simulink model "InverseDynamicsTest"  (R2021b)
settings: Solver=FixedStepAuto  StartTime=0.0  StopTime=5  FixedStep=Ts  RelTol=1e-3
values from neighbouring files (symbols this model uses):
  zdq_A = [1 3*wc 3*wc^2 wc^3]    [search_observer_parameters.m]
  zdq_B = [0 0 0 wc^3]    [search_observer_parameters.m]
undefined symbols (not defined in the file or in its folder): alphas_m, conf, dh, gravity, lambdas_m, x0
libraries: simulink x2, robotcorelib x2, vrlib x1
settings Model: Creator=eros  LastModifiedBy=Sebastiano
settings SolverCC: AlgebraicLoopSolver=TrustRegion
settings DebuggingCC: SFMachineParentedDataDiag=warning

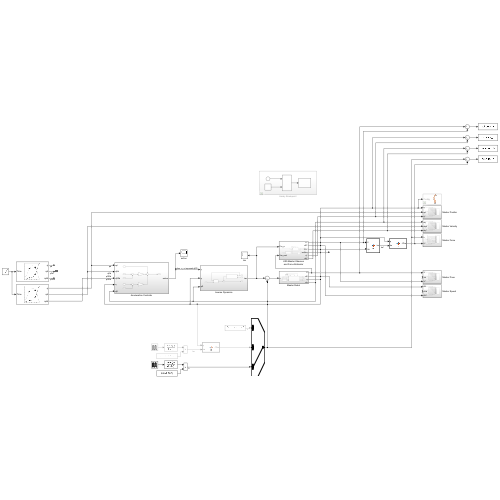
[thumbnail: Simulink's stored preview of the top-level diagram]
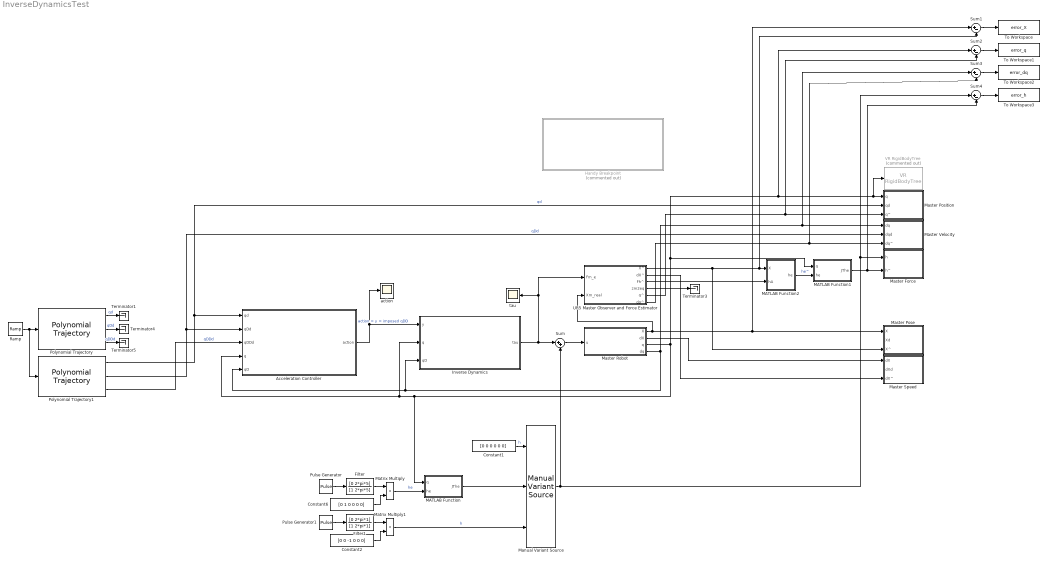
== system InverseDynamicsTest ==
  Acceleration Controller : Subsystem
  Constant1 : Constant  Value=[0 0 0 0 0 0]
  Constant2 : Constant  Value=[0 0 -1 0 0 0]
  Constant6 : Constant  Value=[0 1 0 0 0 0]
  Filter : TransferFcn  Numerator=[0 2*pi*5]  Denominator=[1 2*pi*5]
  Filter1 : TransferFcn  Numerator=[0 2*pi*1]  Denominator=[1 2*pi*1]
  Handy Breakpoint : Subsystem  Commented=on
  Inverse Dynamics : Subsystem
  MATLAB Function : MATLAB Function  TreatAsAtomicUnit=on
  MATLAB Function1 : MATLAB Function  TreatAsAtomicUnit=on
  MATLAB Function2 : MATLAB Function  TreatAsAtomicUnit=on
  Manual Variant Source : simulink/Signal Routing/Manual Variant Source  NumChoices=3  LabelModeActiveChoice=V_3
  Master Force : Subsystem
  Master Pose : Subsystem
  Master Position : Subsystem
  Master Robot : Subsystem
  Master Speed : Subsystem
  Master Velocity : Subsystem
  Matrix Multiply : Product
  Matrix Multiply1 : Product
  Polynomial Trajectory : robotcorelib/Polynomial Trajectory  WaypointSource=Internal  Waypoints=[-1.6007 -1.7271 -2.203 -0.808 1.5951 -0.031; 0 0 0 0 0 0]'  TimePoints=[ 0, 5]  TimeInterval=[ 1, 4 ]  Method=Cubic Polynomial  ParameterSource=Internal  VelocityBoundaryCondition=zeros( 6, 2 )  AccelerationBoundaryCondition=zeros( 2, 5 )  SimulateUsing=Code generation
  Polynomial Trajectory1 : robotcorelib/Polynomial Trajectory  WaypointSource=Internal  Waypoints=[conf.init.q0 conf.init.q0]  TimePoints=[ 0, 5]  TimeInterval=[ 1, 4 ]  Method=Cubic Polynomial  ParameterSource=Internal  VelocityBoundaryCondition=zeros( 6, 2 )  AccelerationBoundaryCondition=zeros( 2, 5 )  SimulateUsing=Code generation
  Pulse Generator : DiscretePulseGenerator  PulseType=Time based  Amplitude=25  Period=3  PulseWidth=50  PhaseDelay=0.5
  Pulse Generator1 : DiscretePulseGenerator  PulseType=Time based  Amplitude=25  Period=3  PulseWidth=50  PhaseDelay=0.5
  Ramp : simulink/Sources/Ramp  slope=1  start=0  InitialOutput=0
  Sum : Sum  Inputs=|++
  Sum{1..4} (4 alike) : Sum  Inputs=|+-
  Terminator{1,3..5} (4 alike) : Terminator
  To Workspace : ToWorkspace  VariableName=error_X  SaveFormat=Timeseries  SampleTime=-1
  To Workspace1 : ToWorkspace  VariableName=error_q  SaveFormat=Timeseries  SampleTime=-1
  To Workspace2 : ToWorkspace  VariableName=error_dq  SaveFormat=Timeseries  SampleTime=-1
  To Workspace3 : ToWorkspace  VariableName=error_h  SaveFormat=Timeseries  SampleTime=-1
  UR5 Master Observer and Force Estimator : Subsystem
  VR RigidBodyTree : vrlib/VR RigidBodyTree  Commented=on  RBT=UR5_robot  useRBT=off  Ts=0.02  ForceViewerOpen=off
      settings: SourceProductBaseCode=SL
  action : Scope
  tau : Scope
  wires:
  Master Robot/4(dq) -> Inverse Dynamics/3(qD), Acceleration Controller/5(qD), Sum3/1, Master Velocity/1(dq)
  Polynomial Trajectory1/3 -> Acceleration Controller/3(qDDd)  "qDDd"
  Inverse Dynamics/1(tau) -> UR5 Master Observer and Force Estimator/1(Fm_e), tau/1, Sum/1
  Polynomial Trajectory1/1 -> Master Position/2(qd), Acceleration Controller/1(qd)  "qd"
  Polynomial Trajectory1/2 -> Master Velocity/2(dqd), Acceleration Controller/2(qDd)  "qDd"
  Acceleration Controller/1(action) -> Inverse Dynamics/1(y), action/1  "action = y = imposed qDD"
  Ramp/1 -> Polynomial Trajectory1/1, Polynomial Trajectory/1
  Sum/1 -> Master Robot/1(u)
  Manual Variant Source/1 -> Sum/2, Sum4/1, Master Force/1(h)
  Pulse Generator/1 -> Filter/1
  Constant6/1 -> Matrix Multiply/2
  Matrix Multiply/1 -> MATLAB Function/2(he)  "he"
  Filter/1 -> Matrix Multiply/1
  UR5 Master Observer and Force Estimator/5(q^) -> Master Position/3(q^), Sum2/2
  UR5 Master Observer and Force Estimator/3(Fh^) -> MATLAB Function2/2(hA)
  UR5 Master Observer and Force Estimator/6(dq^) -> Master Velocity/3(dq^), Sum3/2
  Master Robot/1(X) -> UR5 Master Observer and Force Estimator/2(Xm_real), Sum1/1, Master Pose/1(X)
  Master Robot/2(dX) -> Master Speed/1(dX)
  UR5 Master Observer and Force Estimator/4(zm2eq) -> Terminator3/1
  UR5 Master Observer and Force Estimator/2(dX^) -> Master Speed/3(dX^)
  UR5 Master Observer and Force Estimator/1(X^) -> Master Pose/3(X^), Sum1/2, MATLAB Function2/1(X)
  Constant1/1 -> Manual Variant Source/1  "h"
  MATLAB Function2/1(he) -> MATLAB Function1/2(he)  "he^"
  Master Robot/3(q) -> VR RigidBodyTree/1, Master Position/1(q), Sum2/1, MATLAB Function1/1(q), MATLAB Function/1(q), Acceleration Controller/4(q), Inverse Dynamics/2(q)
  MATLAB Function1/1(JThe) -> Master Force/2(h^), Sum4/2
  MATLAB Function/1(JThe) -> Manual Variant Source/2
  Matrix Multiply1/1 -> Manual Variant Source/3  "h"
  Constant2/1 -> Matrix Multiply1/2
  Filter1/1 -> Matrix Multiply1/1
  Pulse Generator1/1 -> Filter1/1
  Sum1/1 -> To Workspace/1
  Polynomial Trajectory/1 -> Terminator1/1  "qd"
  Polynomial Trajectory/2 -> Terminator4/1  "qDd"
  Polynomial Trajectory/3 -> Terminator5/1  "qDDd"
  Sum2/1 -> To Workspace1/1
  Sum3/1 -> To Workspace2/1
  Sum4/1 -> To Workspace3/1

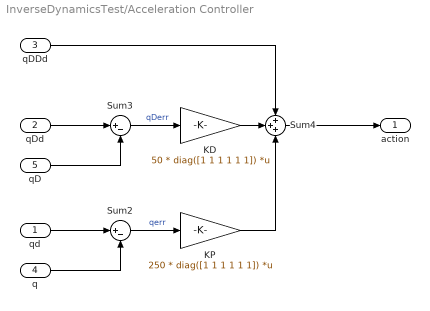
== system InverseDynamicsTest/Acceleration Controller ==
  qd : Inport
  qDd : Inport  Port=2
  qDDd : Inport  Port=3
  q : Inport  Port=4
  qD : Inport  Port=5
  KD : Gain  Gain=50 * diag([1 1 1 1 1 1])  Multiplication=Matrix(K*u) (u vector)
  KP : Gain  Gain=250 * diag([1 1 1 1 1 1])  Multiplication=Matrix(K*u) (u vector)
  Sum2 : Sum  Inputs=|+-
  Sum3 : Sum  Inputs=|+-
  Sum4 : Sum  Inputs=+++
  action : Outport
  wires:
  qDd/1 -> Sum3/1
  KD/1 -> Sum4/2
  KP/1 -> Sum4/3
  qD/1 -> Sum3/2
  Sum3/1 -> KD/1  "qDerr"
  Sum4/1 -> action/1
  Sum2/1 -> KP/1  "qerr"
  qd/1 -> Sum2/1
  qDDd/1 -> Sum4/1
  q/1 -> Sum2/2

== system InverseDynamicsTest/Handy Breakpoint ==
  Assertion : Assertion  AssertionFailFcn=set_param(bdroot,'SimulationCommand','pause')  StopWhenAssertionFail=off
  Clock : Clock
  Constant : Constant  Value=0.5
  Relational Operator : RelationalOperator  Operator=<  OutDataTypeStr=boolean  RndMeth=Simplest
  wires:
  Relational Operator/1 -> Assertion/1
  Constant/1 -> Relational Operator/2
  Clock/1 -> Relational Operator/1

== system InverseDynamicsTest/Inverse Dynamics ==
  y : Inport
  q : Inport  Port=2
  qD : Inport  Port=3
  MATLAB Function : MATLAB Function  TreatAsAtomicUnit=on
  MATLAB Function1 : MATLAB Function  TreatAsAtomicUnit=on
  Sum1 : Sum  Inputs=++|
  tau : Outport
  wires:
  qD/1 -> MATLAB Function/2(qD)
  MATLAB Function/1(n) -> Sum1/1
  MATLAB Function1/1(taud) -> Sum1/2
  q/1 -> MATLAB Function1/1(q), MATLAB Function/1(q)
  y/1 -> MATLAB Function1/2(y)
  Sum1/1 -> tau/1  "tau"

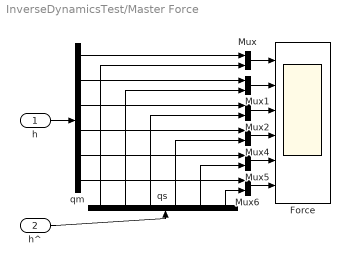
== system InverseDynamicsTest/Master Force ==
  h : Inport
  h^ : Inport  Port=2
  Force : Scope  NumInputPorts=6
  Mux{,1..2,4..6} (6 alike) : Mux  Inputs=2
  qm : Demux  Outputs=dh.dof
  qs : Demux  Outputs=dh.dof
  wires:
  h/1 -> qm/1
  h^/1 -> qs/1
  qm/1 -> Mux/1
  qs/1 -> Mux/2
  qm/2 -> Mux1/1
  qs/2 -> Mux1/2
  qm/3 -> Mux2/1
  qs/3 -> Mux2/2
  qm/4 -> Mux4/1
  qs/4 -> Mux4/2
  Mux/1 -> Force/1
  Mux1/1 -> Force/2
  Mux2/1 -> Force/3
  Mux4/1 -> Force/4
  Mux5/1 -> Force/5
  Mux6/1 -> Force/6
  qs/5 -> Mux5/2
  qm/5 -> Mux5/1
  qm/6 -> Mux6/1
  qs/6 -> Mux6/2

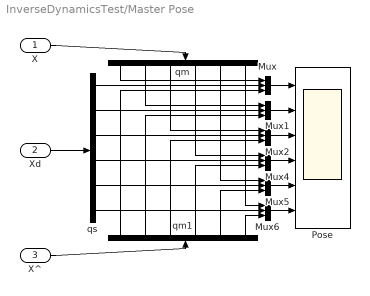
== system InverseDynamicsTest/Master Pose ==
  X : Inport
  Xd : Inport  Port=2
  X^ : Inport  Port=3
  Mux{,1..2,4..6} (6 alike) : Mux  Inputs=3
  Pose : Scope  NumInputPorts=6
  qm : Demux  Outputs=dh.dof
  qm1 : Demux  Outputs=dh.dof
  qs : Demux  Outputs=dh.dof
  wires:
  X/1 -> qm/1
  Xd/1 -> qs/1
  qm/1 -> Mux/1
  qs/1 -> Mux/2
  qm/2 -> Mux1/1
  qs/2 -> Mux1/2
  qm/3 -> Mux2/1
  qs/3 -> Mux2/2
  qm/4 -> Mux4/1
  qs/4 -> Mux4/2
  Mux/1 -> Pose/1
  Mux1/1 -> Pose/2
  Mux2/1 -> Pose/3
  Mux4/1 -> Pose/4
  Mux5/1 -> Pose/5
  Mux6/1 -> Pose/6
  qs/5 -> Mux5/2
  qm/5 -> Mux5/1
  qm/6 -> Mux6/1
  qs/6 -> Mux6/2
  qm1/3 -> Mux2/3
  qm1/2 -> Mux1/3
  qm1/4 -> Mux4/3
  qm1/5 -> Mux5/3
  X^/1 -> qm1/1
  qm1/1 -> Mux/3
  qm1/6 -> Mux6/3

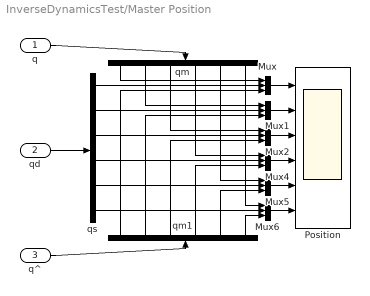
== system InverseDynamicsTest/Master Position ==
  q : Inport
  qd : Inport  Port=2
  q^ : Inport  Port=3
  Mux{,1..2,4..6} (6 alike) : Mux  Inputs=3
  Position : Scope  NumInputPorts=6
  qm : Demux  Outputs=dh.dof
  qm1 : Demux  Outputs=dh.dof
  qs : Demux  Outputs=dh.dof
  wires:
  q/1 -> qm/1
  qd/1 -> qs/1
  qm/1 -> Mux/1
  qs/1 -> Mux/2
  qm/2 -> Mux1/1
  qs/2 -> Mux1/2
  qm/3 -> Mux2/1
  qs/3 -> Mux2/2
  qm/4 -> Mux4/1
  qs/4 -> Mux4/2
  Mux/1 -> Position/1
  Mux1/1 -> Position/2
  Mux2/1 -> Position/3
  Mux4/1 -> Position/4
  Mux5/1 -> Position/5
  Mux6/1 -> Position/6
  qs/5 -> Mux5/2
  qm/5 -> Mux5/1
  qm/6 -> Mux6/1
  qs/6 -> Mux6/2
  qm1/3 -> Mux2/3
  qm1/2 -> Mux1/3
  qm1/4 -> Mux4/3
  qm1/5 -> Mux5/3
  q^/1 -> qm1/1
  qm1/1 -> Mux/3
  qm1/6 -> Mux6/3

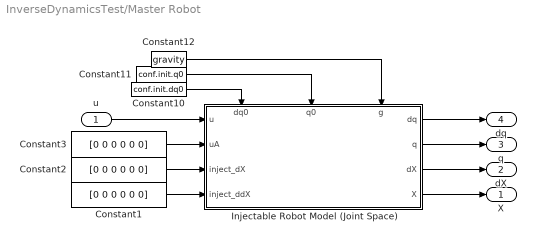
== system InverseDynamicsTest/Master Robot ==
  u : Inport
  Constant1 : Constant  Value=[0 0 0 0 0 0]
  Constant10 : Constant  Value=conf.init.dq0
  Constant11 : Constant  Value=conf.init.q0
  Constant12 : Constant  Value=gravity
  Constant2 : Constant  Value=[0 0 0 0 0 0]
  Constant3 : Constant  Value=[0 0 0 0 0 0]
  Injectable Robot Model (Joint Space) : Subsystem
      settings: PortSchema="{\"entries\":[{\"content\":{\"sides\":[{\"content\":{\"connectorIds\":[\"In1\",\"In2\",\"In3\",\"In4\"]},\"type\":\"ConnectorPlacement.EquallySpacedRectSide\",\"uuid\":\"a8701c64-329e-4144-b882-ecf5d621aff2\"},{\"content\":{\"connectorIds\":[\"Out1\",\"Out2\",\"Out3\",\"Out4\"],\"side\":\"RIGHT\"},\"type\":\"ConnectorPlacement.EquallySpacedRectSide\",\"uuid\":\"4e168703-1cb9-438c-bc6b-9b2d7fbb809e\"},{\"content\":{\"connectorIds\":[\"In5\",\"In6\",\"In7\"],\"side\":\"TOP\"},\"type\":\"ConnectorPlacement.EquallySpacedRectSide\",\"uuid\":\"8fbcb29e-7fab-4224-b4ad-ee01c13d675a\"}]},\"type\":\"ConnectorPlacement.EquallySpacedConnector\",\"uuid\":\"fa721fab-1ce6-4fdf-95fa-8ada3ed2d65c\"}],\"packageUris\":[\"http://schema.mathworks.com/mf0/Connector/R2020b\"],\"version\":\"1.0\"}"
  X : Outport
  dX : Outport  Port=2
  q : Outport  Port=3
  dq : Outport  Port=4
  wires:
  Constant10/1 -> Injectable Robot Model (Joint Space)/5(dq0)
  Constant1/1 -> Injectable Robot Model (Joint Space)/4(inject_ddX)
  Constant11/1 -> Injectable Robot Model (Joint Space)/6(q0)
  Constant2/1 -> Injectable Robot Model (Joint Space)/3(inject_dX)
  Injectable Robot Model (Joint Space)/2(q) -> q/1
  Injectable Robot Model (Joint Space)/3(dX) -> dX/1
  Constant12/1 -> Injectable Robot Model (Joint Space)/7(g)
  Injectable Robot Model (Joint Space)/4(X) -> X/1
  Injectable Robot Model (Joint Space)/1(dq) -> dq/1
  u/1 -> Injectable Robot Model (Joint Space)/1(u)
  Constant3/1 -> Injectable Robot Model (Joint Space)/2(uA)

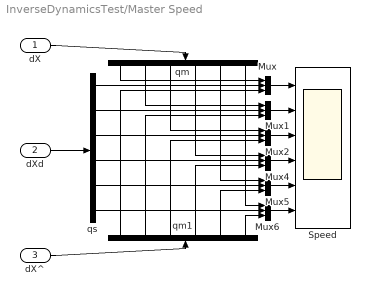
== system InverseDynamicsTest/Master Speed ==
  dX : Inport
  dXd : Inport  Port=2
  dX^ : Inport  Port=3
  Mux{,1..2,4..6} (6 alike) : Mux  Inputs=3
  Speed : Scope  NumInputPorts=6
  qm : Demux  Outputs=dh.dof
  qm1 : Demux  Outputs=dh.dof
  qs : Demux  Outputs=dh.dof
  wires:
  dX/1 -> qm/1
  dXd/1 -> qs/1
  qm/1 -> Mux/1
  qs/1 -> Mux/2
  qm/2 -> Mux1/1
  qs/2 -> Mux1/2
  qm/3 -> Mux2/1
  qs/3 -> Mux2/2
  qm/4 -> Mux4/1
  qs/4 -> Mux4/2
  Mux/1 -> Speed/1
  Mux1/1 -> Speed/2
  Mux2/1 -> Speed/3
  Mux4/1 -> Speed/4
  Mux5/1 -> Speed/5
  Mux6/1 -> Speed/6
  qs/5 -> Mux5/2
  qm/5 -> Mux5/1
  qm/6 -> Mux6/1
  qs/6 -> Mux6/2
  qm1/3 -> Mux2/3
  qm1/2 -> Mux1/3
  qm1/4 -> Mux4/3
  qm1/5 -> Mux5/3
  dX^/1 -> qm1/1
  qm1/1 -> Mux/3
  qm1/6 -> Mux6/3

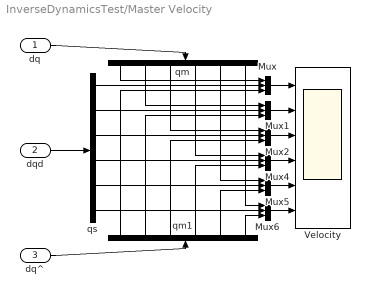
== system InverseDynamicsTest/Master Velocity ==
  dq : Inport
  dqd : Inport  Port=2
  dq^ : Inport  Port=3
  Mux{,1..2,4..6} (6 alike) : Mux  Inputs=3
  Velocity : Scope  NumInputPorts=6
  qm : Demux  Outputs=dh.dof
  qm1 : Demux  Outputs=dh.dof
  qs : Demux  Outputs=dh.dof
  wires:
  dq/1 -> qm/1
  dqd/1 -> qs/1
  qm/1 -> Mux/1
  qs/1 -> Mux/2
  qm/2 -> Mux1/1
  qs/2 -> Mux1/2
  qm/3 -> Mux2/1
  qs/3 -> Mux2/2
  qm/4 -> Mux4/1
  qs/4 -> Mux4/2
  Mux/1 -> Velocity/1
  Mux1/1 -> Velocity/2
  Mux2/1 -> Velocity/3
  Mux4/1 -> Velocity/4
  Mux5/1 -> Velocity/5
  Mux6/1 -> Velocity/6
  qs/5 -> Mux5/2
  qm/5 -> Mux5/1
  qm/6 -> Mux6/1
  qs/6 -> Mux6/2
  qm1/3 -> Mux2/3
  qm1/2 -> Mux1/3
  qm1/4 -> Mux4/3
  qm1/5 -> Mux5/3
  dq^/1 -> qm1/1
  qm1/1 -> Mux/3
  qm1/6 -> Mux6/3

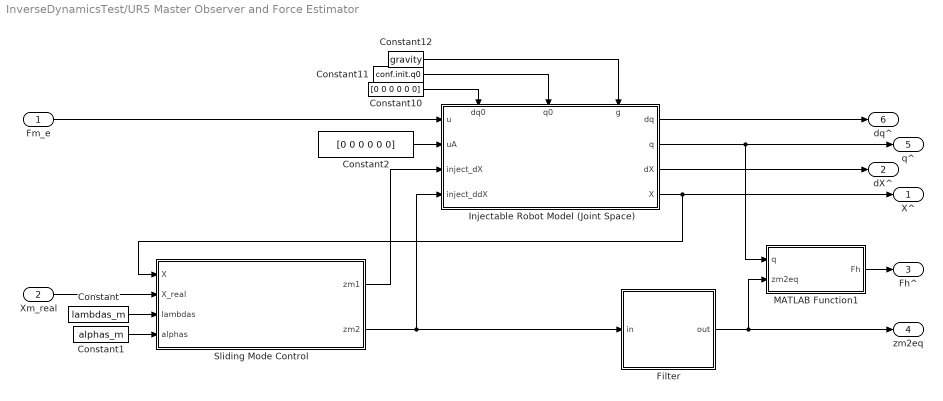
== system InverseDynamicsTest/UR5 Master Observer and Force Estimator ==
  Fm_e : Inport
  Xm_real : Inport  Port=2
  Constant : Constant  Value=lambdas_m
  Constant1 : Constant  Value=alphas_m
  Constant10 : Constant  Value=[0 0 0 0 0 0]
  Constant11 : Constant  Value=conf.init.q0
  Constant12 : Constant  Value=gravity
  Constant2 : Constant  Value=[0 0 0 0 0 0]
  Filter : Subsystem
  Injectable Robot Model (Joint Space) : Subsystem
      settings: PortSchema="{\"entries\":[{\"content\":{\"sides\":[{\"content\":{\"connectorIds\":[\"In1\",\"In2\",\"In3\",\"In4\"]},\"type\":\"ConnectorPlacement.EquallySpacedRectSide\",\"uuid\":\"a8701c64-329e-4144-b882-ecf5d621aff2\"},{\"content\":{\"connectorIds\":[\"Out1\",\"Out2\",\"Out3\",\"Out4\"],\"side\":\"RIGHT\"},\"type\":\"ConnectorPlacement.EquallySpacedRectSide\",\"uuid\":\"4e168703-1cb9-438c-bc6b-9b2d7fbb809e\"},{\"content\":{\"connectorIds\":[\"In5\",\"In6\",\"In7\"],\"side\":\"TOP\"},\"type\":\"ConnectorPlacement.EquallySpacedRectSide\",\"uuid\":\"8fbcb29e-7fab-4224-b4ad-ee01c13d675a\"}]},\"type\":\"ConnectorPlacement.EquallySpacedConnector\",\"uuid\":\"fa721fab-1ce6-4fdf-95fa-8ada3ed2d65c\"}],\"packageUris\":[\"http://schema.mathworks.com/mf0/Connector/R2020b\"],\"version\":\"1.0\"}"
  MATLAB Function1 : MATLAB Function  TreatAsAtomicUnit=on
  Sliding Mode Control : Subsystem
  X^ : Outport
  dX^ : Outport  Port=2
  Fh^ : Outport  Port=3
  zm2eq : Outport  Port=4
  q^ : Outport  Port=5
  dq^ : Outport  Port=6
  wires:
  Filter/1(out) -> MATLAB Function1/2(zm2eq), zm2eq/1
  Sliding Mode Control/1(zm1) -> Injectable Robot Model (Joint Space)/3(inject_dX)
  Sliding Mode Control/2(zm2) -> Injectable Robot Model (Joint Space)/4(inject_ddX), Filter/1(in)
  Constant1/1 -> Sliding Mode Control/4(alphas)
  Constant/1 -> Sliding Mode Control/3(lambdas)
  Xm_real/1 -> Sliding Mode Control/2(X_real)
  Injectable Robot Model (Joint Space)/4(X) -> X^/1, Sliding Mode Control/1(X)
  Injectable Robot Model (Joint Space)/3(dX) -> dX^/1
  Constant11/1 -> Injectable Robot Model (Joint Space)/6(q0)
  Fm_e/1 -> Injectable Robot Model (Joint Space)/1(u)
  Constant10/1 -> Injectable Robot Model (Joint Space)/5(dq0)
  Injectable Robot Model (Joint Space)/1(dq) -> dq^/1
  Constant12/1 -> Injectable Robot Model (Joint Space)/7(g)
  Injectable Robot Model (Joint Space)/2(q) -> MATLAB Function1/1(q), q^/1
  MATLAB Function1/1(Fh) -> Fh^/1
  Constant2/1 -> Injectable Robot Model (Joint Space)/2(uA)

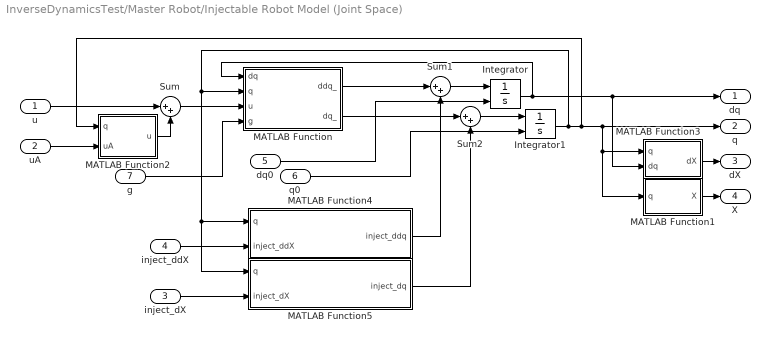
== system InverseDynamicsTest/Master Robot/Injectable Robot Model (Joint Space) ==
  u : Inport
  uA : Inport  Port=2
  inject_dX : Inport  Port=3
  inject_ddX : Inport  Port=4
  dq0 : Inport  Port=5
  q0 : Inport  Port=6
  g : Inport  Port=7
  Integrator : Integrator  InitialConditionSource=external  InitialCondition=x0
  Integrator1 : Integrator  InitialConditionSource=external  InitialCondition=x0
  MATLAB Function : MATLAB Function  TreatAsAtomicUnit=on
  MATLAB Function1 : MATLAB Function  TreatAsAtomicUnit=on
  MATLAB Function2 : MATLAB Function  TreatAsAtomicUnit=on
  MATLAB Function3 : MATLAB Function  TreatAsAtomicUnit=on
  MATLAB Function4 : MATLAB Function  TreatAsAtomicUnit=on
  MATLAB Function5 : MATLAB Function  TreatAsAtomicUnit=on
  Sum : Sum  Inputs=|++
  Sum1 : Sum  Inputs=|++
  Sum2 : Sum  Inputs=|++
  dq : Outport
  q : Outport  Port=2
  dX : Outport  Port=3
  X : Outport  Port=4
  wires:
  g/1 -> MATLAB Function/4(g)
  u/1 -> Sum/1
  dq0/1 -> Integrator/2
  Integrator1/1 -> MATLAB Function2/1(q), q/1, MATLAB Function1/1(q), MATLAB Function3/1(q), MATLAB Function5/1(q), MATLAB Function4/1(q), MATLAB Function/2(q)
  uA/1 -> MATLAB Function2/2(uA)
  MATLAB Function1/1(X) -> X/1
  Integrator/1 -> MATLAB Function3/2(dq), dq/1, MATLAB Function/1(dq)
  MATLAB Function3/1(dX) -> dX/1
  MATLAB Function2/1(u) -> Sum/2
  Sum/1 -> MATLAB Function/3(u)
  MATLAB Function/1(ddq_) -> Sum1/1
  q0/1 -> Integrator1/2
  Sum1/1 -> Integrator/1
  MATLAB Function/2(dq_) -> Sum2/1
  Sum2/1 -> Integrator1/1
  inject_ddX/1 -> MATLAB Function4/2(inject_ddX)
  inject_dX/1 -> MATLAB Function5/2(inject_dX)
  MATLAB Function4/1(inject_ddq) -> Sum1/2
  MATLAB Function5/1(inject_dq) -> Sum2/2

== system InverseDynamicsTest/UR5 Master Observer and Force Estimator/Filter ==
  in : Inport
  Demux : Demux  Outputs=6
  Filter{,1..5} (6 alike) : TransferFcn  Numerator=zdq_B  Denominator=zdq_A
  Mux : Mux  Inputs=6
  out : Outport
  wires:
  Demux/4 -> Filter3/1
  Demux/6 -> Filter5/1
  Demux/2 -> Filter1/1
  Demux/5 -> Filter4/1
  Demux/1 -> Filter/1
  Demux/3 -> Filter2/1
  in/1 -> Demux/1
  Mux/1 -> out/1
  Filter/1 -> Mux/1
  Filter1/1 -> Mux/2
  Filter2/1 -> Mux/3
  Filter3/1 -> Mux/4
  Filter4/1 -> Mux/5
  Filter5/1 -> Mux/6

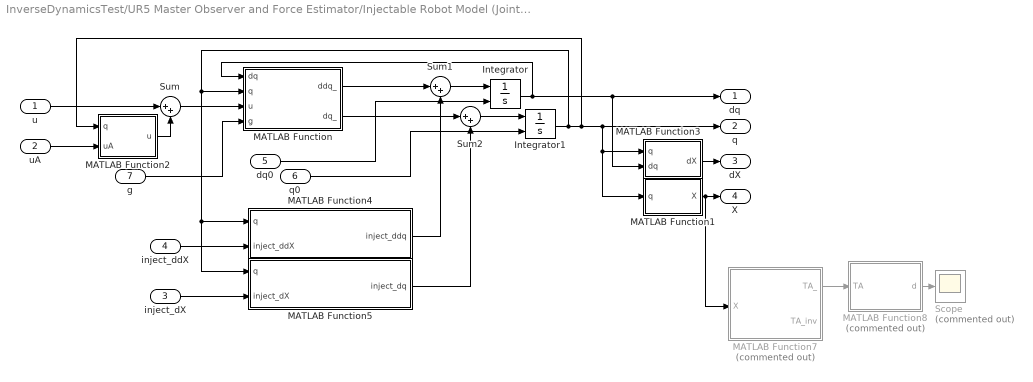
== system InverseDynamicsTest/UR5 Master Observer and Force Estimator/Injectable Robot Model (Joint Space) ==
  u : Inport
  uA : Inport  Port=2
  inject_dX : Inport  Port=3
  inject_ddX : Inport  Port=4
  dq0 : Inport  Port=5
  q0 : Inport  Port=6
  g : Inport  Port=7
  Integrator : Integrator  InitialConditionSource=external  InitialCondition=x0
  Integrator1 : Integrator  InitialConditionSource=external  InitialCondition=x0
  MATLAB Function : MATLAB Function  TreatAsAtomicUnit=on
  MATLAB Function1 : MATLAB Function  TreatAsAtomicUnit=on
  MATLAB Function2 : MATLAB Function  TreatAsAtomicUnit=on
  MATLAB Function3 : MATLAB Function  TreatAsAtomicUnit=on
  MATLAB Function4 : MATLAB Function  TreatAsAtomicUnit=on
  MATLAB Function5 : MATLAB Function  TreatAsAtomicUnit=on
  MATLAB Function7 : MATLAB Function  Commented=on  TreatAsAtomicUnit=on
  MATLAB Function8 : MATLAB Function  Commented=on  TreatAsAtomicUnit=on
  Scope : Scope  Commented=on
  Sum : Sum  Inputs=|++
  Sum1 : Sum  Inputs=|++
  Sum2 : Sum  Inputs=|++
  dq : Outport
  q : Outport  Port=2
  dX : Outport  Port=3
  X : Outport  Port=4
  wires:
  g/1 -> MATLAB Function/4(g)
  u/1 -> Sum/1
  dq0/1 -> Integrator/2
  Integrator1/1 -> MATLAB Function2/1(q), q/1, MATLAB Function1/1(q), MATLAB Function3/1(q), MATLAB Function5/1(q), MATLAB Function4/1(q), MATLAB Function/2(q)
  uA/1 -> MATLAB Function2/2(uA)
  MATLAB Function1/1(X) -> MATLAB Function7/1(X), X/1
  Integrator/1 -> MATLAB Function3/2(dq), dq/1, MATLAB Function/1(dq)
  MATLAB Function3/1(dX) -> dX/1
  MATLAB Function2/1(u) -> Sum/2
  Sum/1 -> MATLAB Function/3(u)
  MATLAB Function/1(ddq_) -> Sum1/1
  q0/1 -> Integrator1/2
  Sum1/1 -> Integrator/1
  MATLAB Function/2(dq_) -> Sum2/1
  Sum2/1 -> Integrator1/1
  inject_ddX/1 -> MATLAB Function4/2(inject_ddX)
  inject_dX/1 -> MATLAB Function5/2(inject_dX)
  MATLAB Function4/1(inject_ddq) -> Sum1/2
  MATLAB Function5/1(inject_dq) -> Sum2/2
  MATLAB Function7/1(TA_) -> MATLAB Function8/1(TA)
  MATLAB Function8/1(d) -> Scope/1

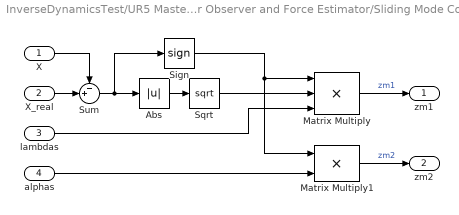
== system InverseDynamicsTest/UR5 Master Observer and Force Estimator/Sliding Mode Control ==
  X : Inport
  X_real : Inport  Port=2
  lambdas : Inport  Port=3
  alphas : Inport  Port=4
  Abs : Abs
  Matrix Multiply : Product  Inputs=***
  Matrix Multiply1 : Product
  Sign : Signum
  Sqrt : Sqrt  SaturateOnIntegerOverflow=on
  Sum : Sum  Inputs=-+|
  zm1 : Outport
  zm2 : Outport  Port=2
  wires:
  Sum/1 -> Sign/1, Abs/1
  Abs/1 -> Sqrt/1
  X/1 -> Sum/1
  lambdas/1 -> Matrix Multiply/3
  Sqrt/1 -> Matrix Multiply/2
  X_real/1 -> Sum/2
  Matrix Multiply/1 -> zm1/1  "zm1"
  Matrix Multiply1/1 -> zm2/1  "zm2"
  alphas/1 -> Matrix Multiply1/2
  Sign/1 -> Matrix Multiply/1, Matrix Multiply1/1

== matlab function InverseDynamicsTest/Inverse Dynamics/MATLAB Function ==
  data: q input; qD input; n output; dh parameter; gravity parameter
function n = n(q, qD, dh, gravity)

    C = C_rne(dh, q, qD);
    G = G_rne(dh, q, gravity);

    n = C * qD + G;

== matlab function InverseDynamicsTest/Master Robot/Injectable Robot Model (Joint Space)/MATLAB Function5 ==
  data: q input size=dh.dof; inject_dq output size=dh.dof; inject_dX input size=6; dh parameter
function inject_dq = get_inject_dq(q, inject_dX, dh)
    JA = JA_rne(dh, q);
    inject_dq = pinv(JA) * inject_dX;
end

== matlab function InverseDynamicsTest/Inverse Dynamics/MATLAB Function1 ==
  data: q input; taud output; y input; dh parameter
function taud = B(q, y, dh)

    B = B_rne(dh, q);

    taud = B*y;

== matlab function InverseDynamicsTest/UR5 Master Observer and Force Estimator/Injectable Robot Model (Joint Space)/MATLAB Function1 ==
  data: X output; q input; dh parameter
function X = K(q, dh)
    X = K_rne(dh, q);
end

== matlab function InverseDynamicsTest/MATLAB Function ==
  data: JThe output; q input; he input; dh parameter
function JThe = JT(q, he, dh)
    JThe = J_rne(dh, q)' * he;
end

== matlab function InverseDynamicsTest/UR5 Master Observer and Force Estimator/Injectable Robot Model (Joint Space)/MATLAB Function7 ==
  data: TA_ output size=[6,6]; X input size=6; TA_inv output size=[6,6]
function [TA_, TA_inv] = TA_X(X)
    TA_ = TA(X);
    TA_inv = pinv(TA_);
end

== matlab function InverseDynamicsTest/UR5 Master Observer and Force Estimator/Injectable Robot Model (Joint Space)/MATLAB Function3 ==
  data: dh parameter; dX output; q input; dq input
function dX = JA(dh, q, dq)
    dX = JA_rne(dh, q)*dq;
end

== matlab function InverseDynamicsTest/UR5 Master Observer and Force Estimator/Injectable Robot Model (Joint Space)/MATLAB Function4 ==
  data: q input size=dh.dof; inject_ddq output size=dh.dof; inject_ddX input size=6; dh parameter
function inject_ddq = get_inject_ddq(q, inject_ddX, dh)
    JA = JA_rne(dh, q);
    inject_ddq = pinv(JA) * inject_ddX;
end

== matlab function InverseDynamicsTest/UR5 Master Observer and Force Estimator/Injectable Robot Model (Joint Space)/MATLAB Function8 ==
  data: TA input; d output
function d = detTA(TA)
    d = det(TA);
end

== matlab function InverseDynamicsTest/Master Robot/Injectable Robot Model (Joint Space)/MATLAB Function ==
  data ddq_ settings: updateMethod=SF_CONTINUOUS_TIME_DATA
  data dq_ settings: updateMethod=SF_CONTINUOUS_TIME_DATA
  data dq settings: updateMethod=SF_CONTINUOUS_TIME_DATA
  data q settings: updateMethod=SF_CONTINUOUS_TIME_DATA
  data u settings: updateMethod=SF_CONTINUOUS_TIME_DATA
  data: ddq_ output size=dh.dof; dq_ output size=dh.dof; dq input size=dh.dof; q input size=dh.dof; u input size=dh.dof; g input size=3; dh parameter
function [ddq_, dq_]  = RobotSystem(dq, q, u, g, dh)
    
    % compute dynamics
    B = B_rne(dh, q);
    C = C_rne(dh, q, dq);
    G = G_rne(dh, q, g);

    dq_ = dq(1:6);

    ddq = B \ (u - C*dq - G);
    ddq_ = ddq(1:6);
end

== matlab function InverseDynamicsTest/MATLAB Function1 ==
  data: JThe output; q input; he input; dh parameter
function JThe = JT(q, he, dh)
    JThe = J_rne(dh, q)' * he;
end

== matlab function InverseDynamicsTest/UR5 Master Observer and Force Estimator/Injectable Robot Model (Joint Space)/MATLAB Function5 ==
  data: q input size=dh.dof; inject_dq output size=dh.dof; inject_dX input size=6; dh parameter
function inject_dq = get_inject_dq(q, inject_dX, dh)
    JA = JA_rne(dh, q);
    inject_dq = pinv(JA) * inject_dX;
end

== matlab function InverseDynamicsTest/Master Robot/Injectable Robot Model (Joint Space)/MATLAB Function1 ==
  data: X output; q input; dh parameter
function X = K(q, dh)
    X = K_rne(dh, q);
end

== matlab function InverseDynamicsTest/UR5 Master Observer and Force Estimator/Injectable Robot Model (Joint Space)/MATLAB Function2 ==
  data: q input; uA input; u output; dh parameter
function u = JAT(q,uA, dh)
    u = JA_rne(dh,q)' * uA;
end

== matlab function InverseDynamicsTest/MATLAB Function2 ==
  data: he output; X input; hA input
function he = TAT_1(X, hA)
    TA_ = TA(X);
    rpinv = (TA_*TA_') \ TA_;
    he = rpinv * hA;
end

== matlab function InverseDynamicsTest/Master Robot/Injectable Robot Model (Joint Space)/MATLAB Function2 ==
  data: q input; uA input; u output; dh parameter
function u = JAT(q,uA, dh)
    u = JA_rne(dh,q)' * uA;
end

== matlab function InverseDynamicsTest/Master Robot/Injectable Robot Model (Joint Space)/MATLAB Function3 ==
  data: dh parameter; dX output; q input; dq input
function dX = JA(dh, q, dq)
    dX = JA_rne(dh, q)*dq;
end

== matlab function InverseDynamicsTest/UR5 Master Observer and Force Estimator/MATLAB Function1 ==
  data: Fh output; q input; zm2eq input; dh parameter
function Fh = BA_zm(q, zm2eq, dh)
     BA = BA_rne(dh, q);
     Fh = BA * zm2eq;
end

== matlab function InverseDynamicsTest/Master Robot/Injectable Robot Model (Joint Space)/MATLAB Function4 ==
  data: q input size=dh.dof; inject_ddq output size=dh.dof; inject_ddX input size=6; dh parameter
function inject_ddq = get_inject_ddq(q, inject_ddX, dh)
    JA = JA_rne(dh, q);
    inject_ddq = pinv(JA) * inject_ddX;
end

== matlab function InverseDynamicsTest/UR5 Master Observer and Force Estimator/Injectable Robot Model (Joint Space)/MATLAB Function ==
  data ddq_ settings: updateMethod=SF_CONTINUOUS_TIME_DATA
  data dq_ settings: updateMethod=SF_CONTINUOUS_TIME_DATA
  data dq settings: updateMethod=SF_CONTINUOUS_TIME_DATA
  data q settings: updateMethod=SF_CONTINUOUS_TIME_DATA
  data u settings: updateMethod=SF_CONTINUOUS_TIME_DATA
  data: ddq_ output size=dh.dof; dq_ output size=dh.dof; dq input size=dh.dof; q input size=dh.dof; u input size=dh.dof; g input size=3; dh parameter
function [ddq_, dq_]  = RobotSystem(dq, q, u, g, dh)
    
    % compute dynamics
    B = B_rne(dh, q);
    C = C_rne(dh, q, dq);
    G = G_rne(dh, q, g);

    dq_ = dq(1:6);

    ddq = B \ (u - C*dq - G);
    ddq_ = ddq(1:6);
end
